simulink model "index"  (R2020a)
settings: Solver=FixedStepAuto  StartTime=0.0  StopTime=10.0  RelTol=1e-3
settings Model: Creator=julius  LastModifiedBy=julius
settings SolverCC: ZeroCrossAlgorithm=Adaptive
settings OptimizationCC: DefaultParameterBehavior=Inlined  OptimizeBlockIOStorage=off  EnhancedBackFolding=on  PassReuseOutputArgsThreshold=0  OptimizeDataStoreBuffers=off  BusAssignmentInplaceUpdate=off
settings DebuggingCC: ParameterTunabilityLossMsg=error  SFUnexpectedBacktrackingDiag=warning  SFNoUnconditionalDefaultTransitionDiag=warning
settings HardwareCC: TargetBitPerPointer=64  TargetBitPerSizeT=64  TargetBitPerPtrDiffT=64  TargetLongLongMode=on  TargetIntDivRoundTo=Zero  TargetEndianess=LittleEndian  TargetWordSize=64  TargetHWDeviceType=MATLAB Host  ProdEqTarget=off
settings SFSimCC: MATLABDynamicMemAlloc=off
settings RTWCC: Description=Rapid Simulation Target  SystemTargetFile=rsim.tlc  TemplateMakefile=rsim_default_tmf  GenerateReport=on  BuildConfiguration=Debug  LaunchReport=on
settings CodeAppCC: ForceParamTrailComments=on  OperatorAnnotations=on  MATLABSourceComments=on  EnableCustomComments=on
settings RSimTargetCC: TargetLangStandard=C99 (ISO)  CombineSignalStateStructs=on  SupportVariableSizeSignals=on  GRTInterface=off

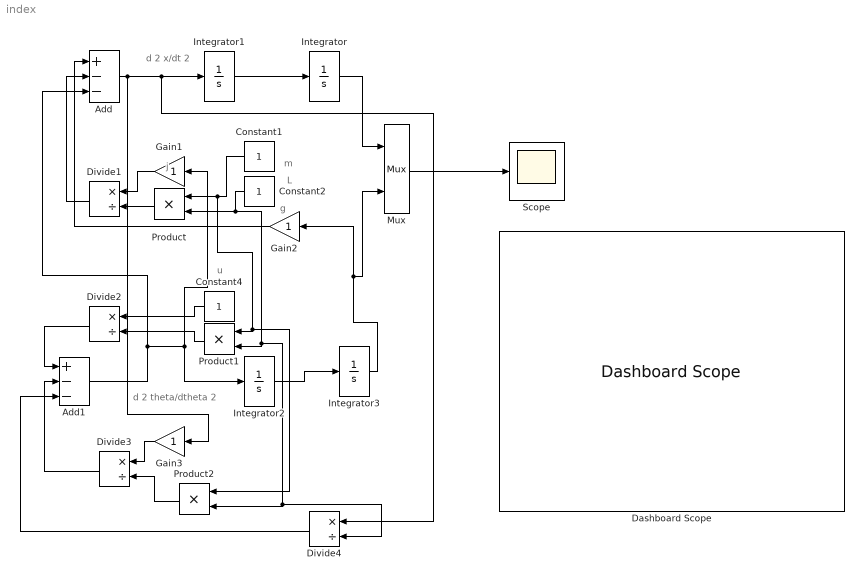
== system index ==
  note: u
  note: L
  note: m
  note: j
  note: g
  note: d 2 theta/dtheta 2
  note: d 2 x/dt 2
  Add : Sum  Inputs=+--
  Add1 : Sum  Inputs=+--
  Constant1 : Constant
  Constant2 : Constant
  Constant4 : Constant
  Dashboard Scope : DashboardScope
  Divide{1..4} (4 alike) : Product  Inputs=*/
  Gain1 : Gain
  Gain2 : Gain
  Gain3 : Gain
  Integrator{,1..3} (4 alike) : Integrator
  Mux : Mux  Inputs=2
  Product : Product
  Product1 : Product
  Product2 : Product
  Scope : Scope
  wires:
  Integrator1/1 -> Integrator/1
  Mux/1 -> Scope/1
  Integrator/1 -> Mux/1
  Add/1 -> Gain3/1, Divide4/1, Integrator1/1
  Add1/1 -> Add/3, Gain1/1, Integrator2/1
  Integrator2/1 -> Integrator3/1
  Integrator3/1 -> Gain2/1, Mux/2
  Gain2/1 -> Add/1
  Gain1/1 -> Divide1/1
  Product/1 -> Divide1/2
  Constant1/1 -> Product2/1, Product1/1, Product/1
  Constant2/1 -> Product/2, Divide4/2, Product2/2, Product1/2
  Divide1/1 -> Add/2
  Divide2/1 -> Add1/1
  Product1/1 -> Divide2/2
  Constant4/1 -> Divide2/1
  Divide3/1 -> Add1/2
  Product2/1 -> Divide3/2
  Gain3/1 -> Divide3/1
  Divide4/1 -> Add1/3
